simulink model "consensus_trans"  (R2023b)
settings: Solver=FixedStepAuto  StartTime=0.0  StopTime=tf  FixedStep=dt  RelTol=1e-3
values from neighbouring files (symbols this model uses):
  A_an = ss_An.A    [red_consensus.m]    (also in red_consensus_2D.m; rendez_vous.m; squared_formation.m; triangular_formation.m)
  alpha = binvar(nt,nr)    [main_red_based_TA.m]    (also in motivating_ex_four.m = 25; old_red_based_TA.m = binvar(nt*nr,1); red_consensus.m = 50; red_consensus_2D.m = 50)
  B = eye(n)    [red_consensus.m]    (also in red_consensus_2D.m = eye(2*n); rendez_vous.m = eye(2*n_t3); squared_formation.m = eye(2*n_t2); squared_formation_dec.m = eye(2*n_t2))
  B_an = ss_An.B    [red_consensus.m]    (also in red_consensus_2D.m; rendez_vous.m; squared_formation.m; triangular_formation.m)
  C = 50    [old_red_based_TA.m]    (also in red_consensus.m = L; red_consensus_2D.m = blkdiag(L,L); rendez_vous.m = blkdiag(Lt3,Lt3); squared_formation.m = blkdiag(Lt2,Lt2))
  C_an = ss_An.C    [red_consensus.m]    (also in red_consensus_2D.m; rendez_vous.m; squared_formation.m; triangular_formation.m)
  C_opt = 1    [motivating_ex_four.m]    (also in red_consensus.m; red_consensus_2D.m = eye(2); rendez_vous.m = eye(2); squared_formation.m = eye(2))
  D_an = ss_An.D    [red_consensus.m]    (also in red_consensus_2D.m; rendez_vous.m; squared_formation.m; triangular_formation.m)
  delta = binvar(nr,1)    [main_red_based_TA.m]    (also in red_consensus.m = [2 1 0 -1 -2 -1  1]'; red_consensus_2D.m = [delta_x;delta_y]; rendez_vous.m = [delta_x_t3;delta_y_t3]; squared_formation.m = [delta_x_t2;delta_y_t2])
  f = 0.2    [consensus.m]    (also in consensus_sat.m; red_consensus.m = 1; red_consensus_2D.m; rendez_vous.m)
  th = 0.05    [motivating_ex_four.m]    (also in red_consensus.m; red_consensus_2D.m; triangular_formation.m)
  u_max = [1,0.5,1,0.4,1.5,0.5,1]'    [red_consensus.m]    (also in red_consensus_2D.m = [u_max_x;u_max_y]; rendez_vous.m = [u_max_x(cc{idx3});u_max_y(cc{idx3})]; squared_formation.m = [u_max_x(cc{idx2});u_max_y(cc{idx2})]; squared_formation_dec.m = [u_max_x(cc{idx2});u_max_y(cc{idx2})])
  x0 = zeros(na,1)    [main_red_based_TA.m]    (also in red_consensus.m = zeros(n,1); red_consensus_2D.m = zeros(n,1); rendez_vous.m = x0_cc3; squared_formation.m = x0_cc2)
  x_an0 = zeros(max(size(A_an)),1)    [red_consensus.m]    (also in red_consensus_2D.m; rendez_vous.m; squared_formation.m; squared_formation_dec.m = zeros(max(size(A_an_n2)),1))
  x_opt0 = 0    [red_consensus.m]    (also in red_consensus_2D.m = zeros(2,1); rendez_vous.m = zeros(2,1); squared_formation.m = zeros(2,1); squared_formation_dec.m = zeros(2,1))
  y0 = zeros(na,1)    [main_red_based_TA.m]    (also in red_consensus_2D.m = zeros(n,1); rendez_vous.m = y0_cc3; squared_formation.m = y0_cc2; triangular_formation.m = y0_cc1)
settings Model: Creator=lorenzo  LastModifiedBy=lorenzo
settings SolverCC: ZeroCrossControl=DisableAll
settings DebuggingCC: IgnoredZcDiagnostic=none

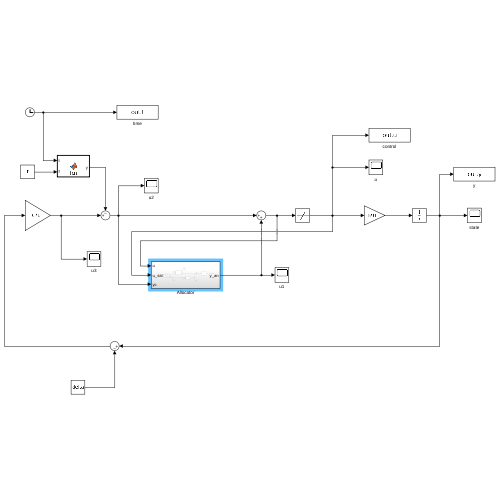
[thumbnail: Simulink's stored preview of the top-level diagram]
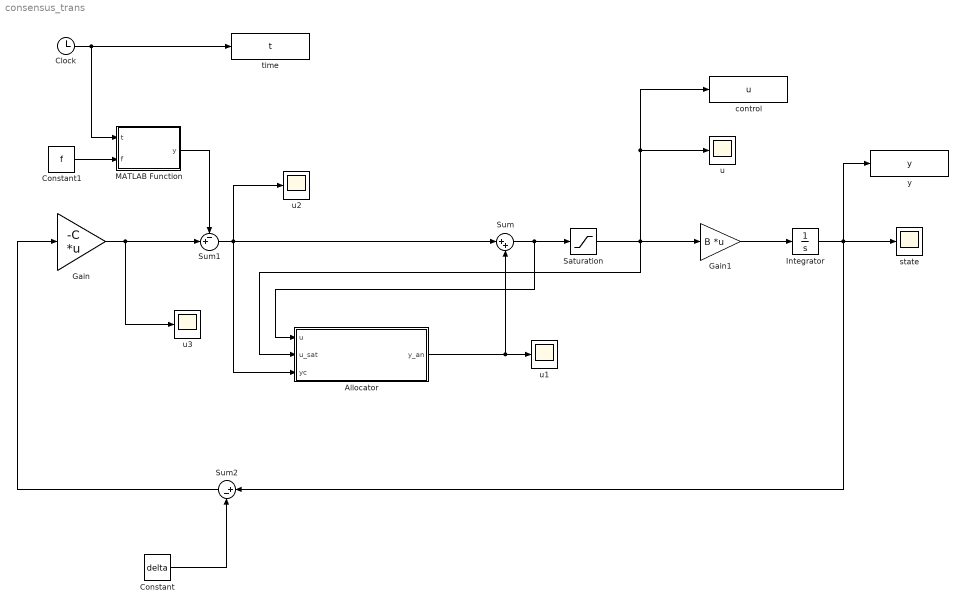
== system consensus_trans ==
  Allocator : Subsystem
  Clock : Clock
  Constant : Constant  Value=delta  VectorParams1D=off
  Constant1 : Constant  Value=f  VectorParams1D=off
  Gain : Gain  Gain=-C  Multiplication=Matrix(K*u)
  Gain1 : Gain  Gain=B  Multiplication=Matrix(K*u)
  Integrator : Integrator  InitialCondition=[x0;y0]
  MATLAB Function : MATLAB Function  TreatAsAtomicUnit=on
  Saturation : Saturate  UpperLimit=u_max  LowerLimit=-u_max
  Sum : Sum  Inputs=|++
  Sum1 : Sum  Inputs=-+|
  Sum2 : Sum  Inputs=|+-
  control : ToWorkspace  VariableName=u  SampleTime=-1
  state : Scope
  time : ToWorkspace  VariableName=t  SampleTime=-1
  u{,1..3} (4 alike) : Scope
  y : ToWorkspace  VariableName=y  SampleTime=-1
  wires:
  Clock/1 -> MATLAB Function/1(t), time/1
  Integrator/1 -> Sum2/1, y/1, state/1
  Sum/1 -> Allocator/1(u), Saturation/1
  Allocator/1(y_an) -> u1/1, Sum/2
  Saturation/1 -> control/1, u/1, Gain1/1, Allocator/2(u_sat)
  Gain1/1 -> Integrator/1
  MATLAB Function/1(y) -> Sum1/1
  Gain/1 -> u3/1, Sum1/2
  Sum1/1 -> u2/1, Allocator/3(yc), Sum/1
  Constant/1 -> Sum2/2
  Sum2/1 -> Gain/1
  Constant1/1 -> MATLAB Function/2(f)

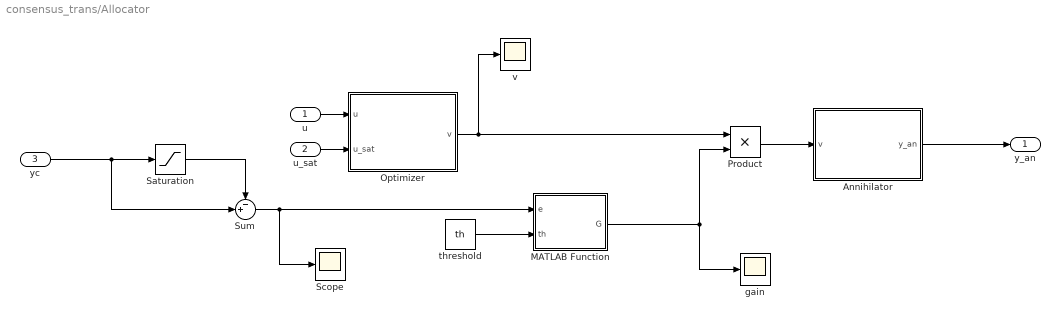
== system consensus_trans/Allocator ==
  u : Inport
  u_sat : Inport  Port=2
  yc : Inport  Port=3
  Annihilator : Subsystem
  MATLAB Function : MATLAB Function  TreatAsAtomicUnit=on
  Optimizer : Subsystem
  Product : Product
  Saturation : Saturate  UpperLimit=u_max  LowerLimit=-u_max
  Scope : Scope
  Sum : Sum  Inputs=-+|
  gain : Scope
  threshold : Constant  Value=th
  v : Scope
  y_an : Outport
  wires:
  threshold/1 -> MATLAB Function/2(th)
  Optimizer/1(v) -> Product/1, v/1
  u_sat/1 -> Optimizer/2(u_sat)
  MATLAB Function/1(G) -> gain/1, Product/2
  u/1 -> Optimizer/1(u)
  Annihilator/1(y_an) -> y_an/1
  Product/1 -> Annihilator/1(v)
  Saturation/1 -> Sum/1
  Sum/1 -> Scope/1, MATLAB Function/1(e)
  yc/1 -> Sum/2, Saturation/1

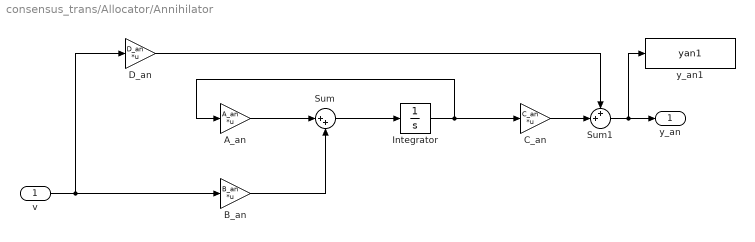
== system consensus_trans/Allocator/Annihilator ==
  v : Inport
  A_an : Gain  Gain=A_an  Multiplication=Matrix(K*u) (u vector)
  B_an : Gain  Gain=B_an  Multiplication=Matrix(K*u) (u vector)
  C_an : Gain  Gain=C_an  Multiplication=Matrix(K*u) (u vector)
  D_an : Gain  Gain=D_an  Multiplication=Matrix(K*u) (u vector)
  Integrator : Integrator  InitialCondition=x_an0
  Sum : Sum  Inputs=|++
  Sum1 : Sum  Inputs=++|
  y_an1 : ToWorkspace  VariableName=yan1  SampleTime=-1
  y_an : Outport
  wires:
  Integrator/1 -> C_an/1, A_an/1
  B_an/1 -> Sum/2
  A_an/1 -> Sum/1
  v/1 -> D_an/1, B_an/1
  Sum/1 -> Integrator/1
  C_an/1 -> Sum1/2
  D_an/1 -> Sum1/1
  Sum1/1 -> y_an1/1, y_an/1

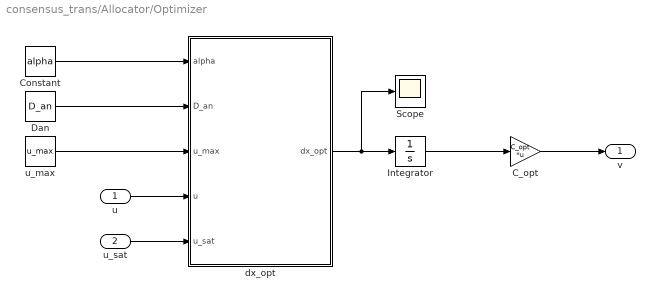
== system consensus_trans/Allocator/Optimizer ==
  u : Inport
  u_sat : Inport  Port=2
  C_opt : Gain  Gain=C_opt  Multiplication=Matrix(K*u) (u vector)
  Constant : Constant  Value=alpha
  Dan : Constant  Value=D_an  VectorParams1D=off
  Integrator : Integrator  InitialCondition=x_opt0
  Scope : Scope
  dx_opt : MATLAB Function  TreatAsAtomicUnit=on
  u_max : Constant  Value=u_max
  v : Outport
  wires:
  dx_opt/1(dx_opt) -> Scope/1, Integrator/1
  C_opt/1 -> v/1
  Constant/1 -> dx_opt/1(alpha)
  Dan/1 -> dx_opt/2(D_an)
  u_max/1 -> dx_opt/3(u_max)
  u/1 -> dx_opt/4(u)
  u_sat/1 -> dx_opt/5(u_sat)
  Integrator/1 -> C_opt/1

== matlab function consensus_trans/MATLAB Function ==
  data: t input; y output; f input
function y = fcn(t,f)

y = [cos(f*t)*ones(7,1);sin(f*t)*ones(7,1)];

== matlab function consensus_trans/Allocator/MATLAB Function ==
  data: e input; G output; th input
function G = fcn(e,th)
norm(e);
eps = th/2;

G=1;

if ( norm(e) < th-eps )
    G = 0;
end
if ( norm(e) > th )
    G = 1;
end
if ( norm(e) <= th && norm(e) >= th-eps )
    G = -2*((norm(e)-(th-eps))/eps)^3+3*((norm(e)-(th-eps))/eps)^2;
end

== matlab function consensus_trans/Allocator/Optimizer/dx_opt ==
  data: dx_opt output; alpha input; D_an input; u_max input; u input; u_sat input
function dx_opt = opt_dyn(alpha,D_an,u_max,u,u_sat)

u1_max = u_max(1);
u2_max = u_max(2);
u3_max = u_max(3);
u4_max = u_max(4);
u5_max = u_max(5);
u6_max = u_max(6);
u7_max = u_max(7);

u11_max = u_max(8);
u22_max = u_max(9);
u33_max = u_max(10);
u44_max = u_max(11);
u55_max = u_max(12);
u66_max = u_max(13);
u77_max = u_max(14);

phi = u - u_sat;

par_der = diag([dsat(u(1),u1_max,0.01), ...
                dsat(u(2),u2_max,0.01), ...
                dsat(u(3),u3_max,0.01), ...
                dsat(u(4),u4_max,0.01), ...
                dsat(u(5),u5_max,0.01), ...
                dsat(u(6),u6_max,0.01), ...
                dsat(u(7),u7_max,0.01), ...
                dsat(u(8),u11_max,0.01), ...
                dsat(u(9),u22_max,0.01), ...
                dsat(u(10),u33_max,0.01), ...
                dsat(u(11),u44_max,0.01), ...
                dsat(u(12),u55_max,0.01), ...
                dsat(u(13),u66_max,0.01), ...
                dsat(u(14),u77_max,0.01),]); 

grad = phi'*(D_an-par_der*D_an);

dx_opt = -alpha*grad';


% phi = yc+Wan0*x_opt;
% 
% %ss_sat = phi;
% 
% %ss_sat = [u1_max * 2/pi * atan(phi(1));u2_max * 2/pi * atan(phi(2))]; 
% 
% ss_sat = [u1_max * tanh(phi(1));u2_max * tanh(phi(2))]; 
% 
% % if ( abs(phi(1))>=u1_max )
% %     ss_sat(1) = sign(phi(1))*u1_max;
% % end
% % if ( abs(phi(2))>=u2_max )
% %     ss_sat(2) = sign(phi(2))*u2_max;
% % end
% 
% %par_der = diag([(u1_max*2/pi)/(1+(phi(1))^2),(u2_max*2/pi)/(1+(phi(2))^2)]);
% 
% par_der = diag([u1_max/(cosh(phi(1)))^2,u2_max/(cosh(phi(2)))^2]);
% 
% %par_der = diag([dsat(phi(1),u1_max,0.01),dsat(phi(2),u2_max,0.01)]); 
% 
% %grad = (yc+Wan0*x_opt-u_sat)'*(Wan0-par_der*Wan0);
% 
% grad = (yc+Wan0*x_opt-ss_sat)'*(Wan0-par_der*Wan0);
% 
% dx_opt = -alpha*grad;
